simulink model "dt_crff2_non_ideal"  (R2025b)
settings: Solver=VariableStepAuto  StartTime=0.0  StopTime=10.0  RelTol=1e-3
undefined symbols (not defined in the file): Fs, k01, K01, k02, K02, k03, K03, k04, K04, k05, K05, k06, K06, k07, K07, k08, K08, k09, K09, k10, K10, k11, K11, k12, K12, k13, K13, k14, K14, k15, K15, k16, K16, k17, K17, k18, K18, k19, K19, k20, K20, k21, K21, k22, K22, k23, K23, k24, K24, k25, K25, k26, K26, k27, K27, k28, K28, k29, K29, k30 ... (+66)
libraries: msbAdcMeasurements x1, cstblocks x1, dspobslib x1
settings Model: Creator=divya  LastModifiedBy=divya

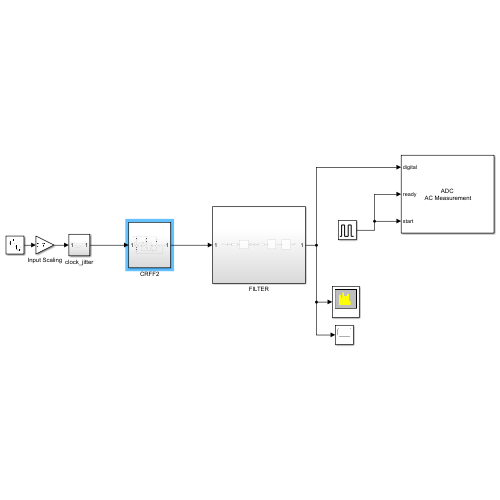
[thumbnail: Simulink's stored preview of the top-level diagram]
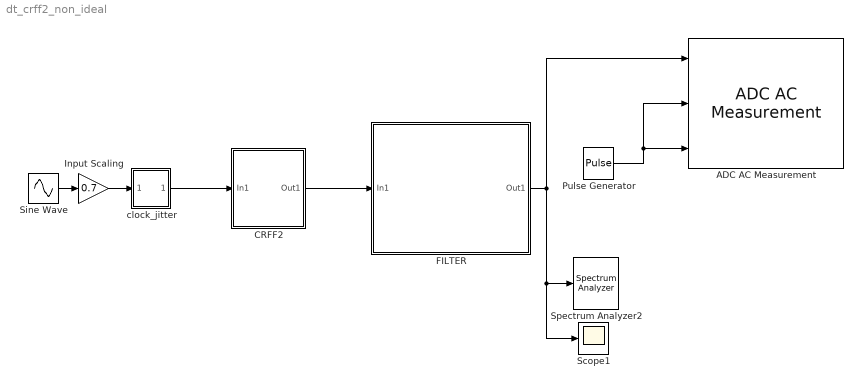
== system dt_crff2_non_ideal ==
  ADC AC Measurement : msbAdcMeasurements/ADC AC Measurement  DistortionMeasurement=Harmonic  InputFrequency=100  Method=Filter bank (slower, requires extra simulation time)  RBW=0.48828  AutoSetRBW=on  NBits=18  Frequency=512e3/1024  HoldOffTime=0  OutputToWorkspace=on  VariableName=adc_ac_out  ShowSpectrum=on
      link override ADC AC Measurement/ADC AC Measurement Spectrum Analyzer: YLimits=[-1125000 -875000]
  CRFF2 : Subsystem
  FILTER : Subsystem
  Input Scaling : Gain  Gain=0.7
  Pulse Generator : DiscretePulseGenerator  PulseType=Time based  Period=1/1e3  PulseWidth=50
  Scope1 : Scope
      settings: ActiveDisplayYMinimum=-1.8E-8  ActiveDisplayYMaximum=1.8E-8
  Sine Wave : Sin  Amplitude=0.5  Frequency=628  SampleTime=1/512e3
  Spectrum Analyzer2 : SpectrumAnalyzer  WindowPosition=[1.000000,1.000000,1536.000000,841.000000,]  ScopeFrameLocation=window  PlotAsTwoSidedSpectrum=off  YLimits=[-207.6433 -122.1238]  SelectedToolstripTab=spectrumAnalyzerToolstrip.spectrumTab
  clock_jitter : Subsystem
  wires:
  CRFF2/1(Out1) -> FILTER/1(In1)
  clock_jitter/1(Out1) -> CRFF2/1(In1)
  Pulse Generator/1 -> ADC AC Measurement/3, ADC AC Measurement/2
  Input Scaling/1 -> clock_jitter/1(In1)
  FILTER/1(Out1) -> ADC AC Measurement/1, Scope1/1, Spectrum Analyzer2/1
  Sine Wave/1 -> Input Scaling/1

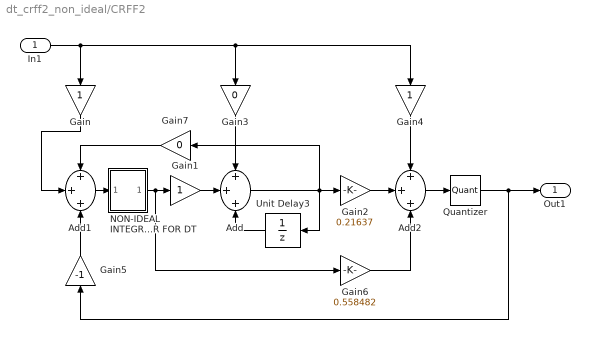
== system dt_crff2_non_ideal/CRFF2 ==
  In1 : Inport
  Add : Sum  RequirementInfo={} %GIDa_3c5f622a_b94f_44a6_8cf5_4d620276e7c1  Inputs=+++
  Add1 : Sum  RequirementInfo={} %GIDa_2560f21a_28c6_47ea_a0df_4ad0b40fcbe5  Inputs=+++
  Add2 : Sum  RequirementInfo={} %GIDa_8d62e077_71f1_449a_b76b_2bda6cdf909d  Inputs=+++
  Gain : Gain  RequirementInfo={} %GIDa_ad436a21_f5dd_4e55_a482_890f0f126b90
  Gain1 : Gain  RequirementInfo={} %GIDa_c3b20c88_4060_4312_8646_d3b95ed7ab58
  Gain2 : Gain  RequirementInfo={} %GIDa_e70bd45e_24a6_44be_901f_827768984ba0  Gain=0.21637
  Gain3 : Gain  RequirementInfo={} %GIDa_dd2b615f_3e17_4946_afe5_8b8154edc31d  Gain=0
  Gain4 : Gain  RequirementInfo={} %GIDa_6be3646e_fc84_4f83_a120_e64b39dc9dcc
  Gain5 : Gain  RequirementInfo={} %GIDa_626d9d2e_4885_4ec0_a1ca_3018a1e5cf17  Gain=-1
  Gain6 : Gain  RequirementInfo={} %GIDa_3141b0aa_4885_4fd5_b8bf_797217bb3f0f  Gain=0.558482
  Gain7 : Gain  RequirementInfo={} %GIDa_7d31512d_d1b8_464e_a954_aed416029a99  Gain=0
  NON-IDEAL INTEGRATOR FOR DT : Subsystem
  Quantizer : Quantizer  RequirementInfo={} %GIDa_4572926b_fdfc_440d_bb41_09360aa605ce  QuantizationInterval=0.25
  Unit Delay3 : UnitDelay  SampleTime=1/(48e3*64)  HasFrameUpgradeWarning=on
  Out1 : Outport
  wires:
  Gain4/1 -> Add2/1
  Gain1/1 -> Add/2
  Add1/1 -> NON-IDEAL INTEGRATOR FOR DT/1(In2)
  Gain3/1 -> Add/1
  Gain5/1 -> Add1/3
  Gain2/1 -> Add2/2
  Unit Delay3/1 -> Add/3
  Gain7/1 -> Add1/1
  Quantizer/1 -> Out1/1, Gain5/1
  Add2/1 -> Quantizer/1
  Add/1 -> Unit Delay3/1, Gain7/1, Gain2/1
  In1/1 -> Gain/1, Gain3/1, Gain4/1
  NON-IDEAL INTEGRATOR FOR DT/1(Out1) -> Gain6/1, Gain1/1
  Gain6/1 -> Add2/3
  Gain/1 -> Add1/2

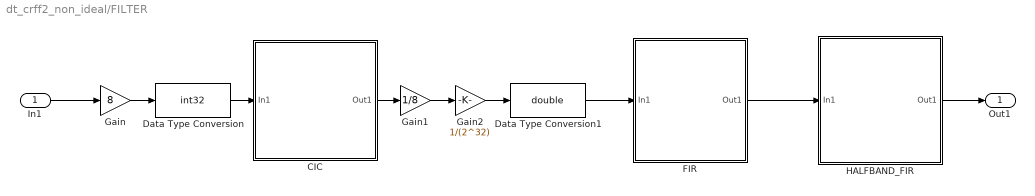
== system dt_crff2_non_ideal/FILTER ==
  In1 : Inport
  CIC : Subsystem
  Data Type Conversion : DataTypeConversion  OutDataTypeStr=int32  SaturateOnIntegerOverflow=off  RndMeth=Floor
  Data Type Conversion1 : DataTypeConversion  OutDataTypeStr=double  SaturateOnIntegerOverflow=off  RndMeth=Floor
  FIR : Subsystem
  Gain : Gain  Gain=8
  Gain1 : Gain  Gain=1/8
  Gain2 : Gain  Gain=1/(2^32)
  HALFBAND_FIR : Subsystem
  Out1 : Outport
  wires:
  Gain2/1 -> Data Type Conversion1/1
  Gain1/1 -> Gain2/1
  Data Type Conversion/1 -> CIC/1(In1)
  CIC/1(Out1) -> Gain1/1
  Gain/1 -> Data Type Conversion/1
  FIR/1(Out1) -> HALFBAND_FIR/1(In1)
  In1/1 -> Gain/1
  Data Type Conversion1/1 -> FIR/1(In1)
  HALFBAND_FIR/1(Out1) -> Out1/1

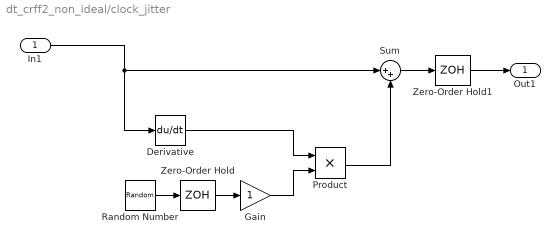
== system dt_crff2_non_ideal/clock_jitter ==
  In1 : Inport
  Derivative : Derivative
  Gain : Gain
  Product : Product
  Random Number : RandomNumber  SampleTime=0.1
  Sum : Sum  Inputs=|++
  Zero-Order Hold : ZeroOrderHold  SampleTime=-1
  Zero-Order Hold1 : ZeroOrderHold  SampleTime=-1
  Out1 : Outport
  wires:
  In1/1 -> Derivative/1, Sum/1
  Derivative/1 -> Product/1
  Zero-Order Hold1/1 -> Out1/1
  Sum/1 -> Zero-Order Hold1/1
  Random Number/1 -> Zero-Order Hold/1
  Product/1 -> Sum/2
  Zero-Order Hold/1 -> Gain/1
  Gain/1 -> Product/2

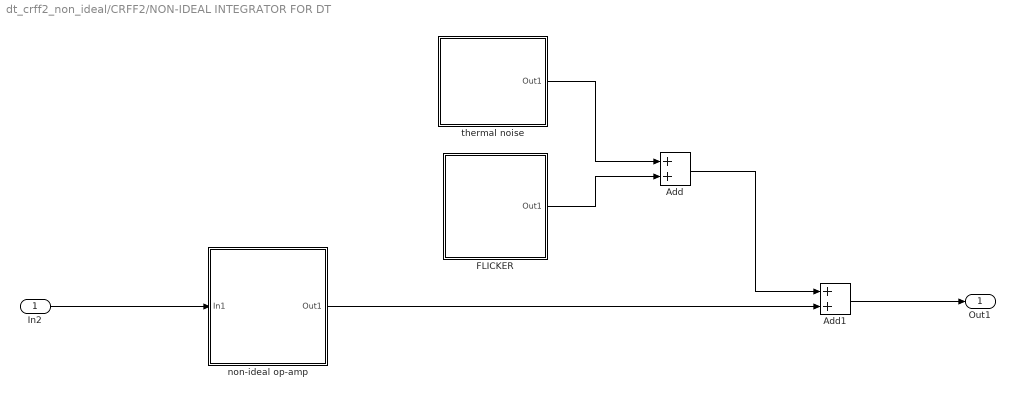
== system dt_crff2_non_ideal/CRFF2/NON-IDEAL INTEGRATOR FOR DT ==
  In2 : Inport
  Add : Sum
  Add1 : Sum
  FLICKER : Subsystem
  "non-ideal op-amp " : Subsystem
  thermal noise : Subsystem
  Out1 : Outport
  wires:
  In2/1 -> "non-ideal op-amp "/1(In1)
  Add/1 -> Add1/1
  Add1/1 -> Out1/1
  "non-ideal op-amp "/1(Out1) -> Add1/2
  thermal noise/1(Out1) -> Add/1
  FLICKER/1(Out1) -> Add/2

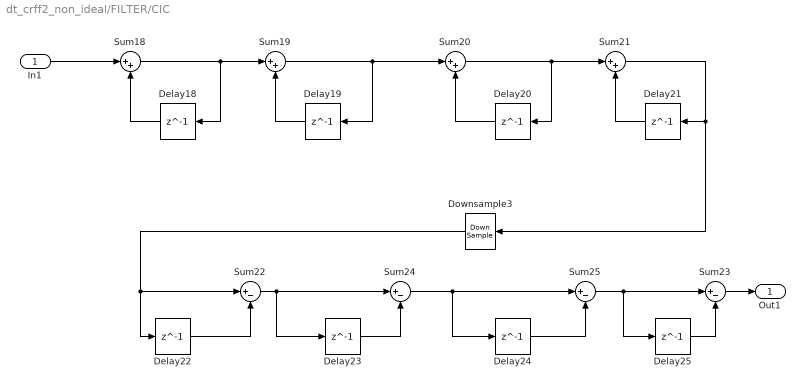
== system dt_crff2_non_ideal/FILTER/CIC ==
  In1 : Inport
  Delay{18..25} (8 alike) : Delay  DelayLength=1  InputProcessing=Columns as channels (frame based)
  Downsample3 : DownSample  N=128  RateOptions=Allow multirate processing
  Sum{18..21} (4 alike) : Sum  Inputs=|++
  Sum{22..25} (4 alike) : Sum  Inputs=|+-
  Out1 : Outport
  wires:
  Downsample3/1 -> Sum22/1, Delay22/1
  Sum19/1 -> Delay19/1, Sum20/1
  Sum20/1 -> Delay20/1, Sum21/1
  Sum22/1 -> Delay23/1, Sum24/1
  Delay24/1 -> Sum25/2
  Sum24/1 -> Delay24/1, Sum25/1
  In1/1 -> Sum18/1
  Sum18/1 -> Delay18/1, Sum19/1
  Delay18/1 -> Sum18/2
  Sum25/1 -> Delay25/1, Sum23/1
  Delay20/1 -> Sum20/2
  Delay22/1 -> Sum22/2
  Delay21/1 -> Sum21/2
  Sum21/1 -> Downsample3/1, Delay21/1
  Delay23/1 -> Sum24/2
  Delay19/1 -> Sum19/2
  Delay25/1 -> Sum23/2
  Sum23/1 -> Out1/1

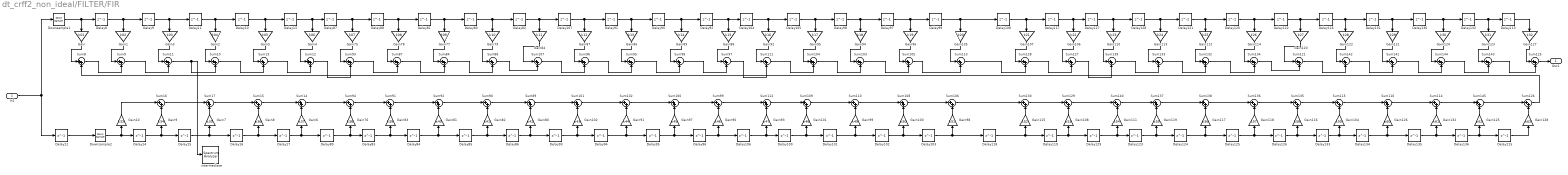
== system dt_crff2_non_ideal/FILTER/FIR ==
  In1 : Inport
  Delay{8..17,80..108,113,115..136} (62 alike) : Delay  DelayLength=1  InputProcessing=Columns as channels (frame based)
  Downsample1 : DownSample  N=4  RateOptions=Allow multirate processing
  Downsample2 : DownSample  N=4  RateOptions=Allow multirate processing
  Gain : Gain  Gain=k01
  Gain1 : Gain  Gain=k02
  Gain10 : Gain  Gain=k33
  Gain100 : Gain  Gain=k50
  Gain101 : Gain  Gain=k48
  Gain102 : Gain  Gain=k43
  Gain104 : Gain  Gain=k59
  Gain105 : Gain  Gain=k20
  Gain106 : Gain  Gain=k22
  Gain107 : Gain  Gain=k21
  Gain108 : Gain  Gain=k53
  Gain110 : Gain  Gain=k23
  Gain111 : Gain  Gain=k54
  Gain112 : Gain  Gain=k25
  Gain113 : Gain  Gain=k24
  Gain114 : Gain  Gain=k26
  Gain115 : Gain  Gain=k52
  Gain116 : Gain  Gain=k58
  Gain117 : Gain  Gain=k56
  Gain118 : Gain  Gain=k57
  Gain119 : Gain  Gain=k55
  Gain120 : Gain  Gain=k27
  Gain121 : Gain  Gain=k29
  Gain122 : Gain  Gain=k28
  Gain123 : Gain  Gain=k31
  Gain124 : Gain  Gain=k30
  Gain125 : Gain  Gain=k62
  Gain126 : Gain  Gain=k60
  Gain127 : Gain  Gain=k32
  Gain128 : Gain  Gain=k63
  Gain132 : Gain  Gain=k61
  Gain2 : Gain  Gain=k04
  Gain3 : Gain  Gain=k03
  Gain4 : Gain  Gain=k06
  Gain5 : Gain  Gain=k05
  Gain6 : Gain  Gain=k37
  Gain7 : Gain  Gain=k35
  Gain75 : Gain  Gain=k07
  Gain76 : Gain  Gain=k38
  Gain77 : Gain  Gain=k09
  Gain78 : Gain  Gain=k08
  Gain79 : Gain  Gain=k10
  Gain8 : Gain  Gain=k36
  Gain80 : Gain  Gain=k42
  Gain81 : Gain  Gain=k40
  Gain82 : Gain  Gain=k41
  Gain83 : Gain  Gain=k39
  Gain84 : Gain  Gain=k11
  Gain86 : Gain  Gain=k13
  Gain87 : Gain  Gain=k12
  Gain88 : Gain  Gain=k15
  Gain89 : Gain  Gain=k14
  Gain9 : Gain  Gain=k34
  Gain90 : Gain  Gain=k46
  Gain91 : Gain  Gain=k44
  Gain92 : Gain  Gain=k16
  Gain93 : Gain  Gain=k47
  Gain94 : Gain  Gain=k18
  Gain95 : Gain  Gain=k17
  Gain96 : Gain  Gain=k19
  Gain97 : Gain  Gain=k45
  Gain98 : Gain  Gain=k51
  Gain99 : Gain  Gain=k49
  Sum{8..17,84,87..116,121,125..130,132..145} (62 alike) : Sum  Inputs=|++
  intermediate : SpectrumAnalyzer  WindowPosition=[1.000000,1.000000,1536.000000,841.000000,]  ScopeFrameLocation=window  Span=1000  StartFrequency=-500  StopFrequency=500  YLimits=[-211.6942 -128.1697]
  Out1 : Outport
  wires:
  Sum107/1 -> Sum96/2
  Delay104/1 -> Delay105/1, Gain92/1
  Delay88/1 -> Gain78/1, Delay81/1
  Sum98/1 -> Sum97/2
  Gain132/1 -> Sum114/2
  Sum135/1 -> Sum115/1
  Downsample1/1 -> Delay8/1, Gain/1
  Gain80/1 -> Sum89/2
  Delay84/1 -> Delay85/1, Gain81/1
  Gain120/1 -> Sum121/1
  Sum142/1 -> Sum141/2
  Sum96/1 -> Sum95/2
  Delay108/1 -> Gain107/1, Delay117/1
  Delay92/1 -> Delay104/1, Gain88/1
  Sum100/1 -> Sum99/1
  Sum94/1 -> Sum91/1
  Delay129/1 -> Gain111/1, Delay123/1
  Gain116/1 -> Sum135/2
  Delay81/1 -> Delay80/1, Gain77/1
  Delay132/1 -> Delay113/1, Gain123/1
  Delay101/1 -> Delay102/1, Gain99/1
  Sum137/1 -> Sum138/1
  Gain96/1 -> Sum105/1
  Delay125/1 -> Gain118/1, Delay126/1
  Delay116/1 -> Delay131/1, Gain122/1
  Delay97/1 -> Gain96/1, Delay99/1
  Downsample2/1 -> Gain10/1, Delay14/1
  Delay80/1 -> Delay82/1, Gain79/1
  Gain111/1 -> Sum140/2
  Gain2/1 -> Sum10/1
  Sum17/1 -> Sum15/1
  Gain118/1 -> Sum136/2
  Delay89/1 -> Gain76/1, Delay83/1
  Sum126/1 -> Sum8/2
  Gain123/1 -> Sum143/1
  Delay113/1 -> Gain127/1
  Sum92/1 -> Sum90/1
  Gain100/1 -> Sum108/2
  Sum10/1 -> Sum13/2
  Gain3/1 -> Sum11/1
  Delay122/1 -> Gain120/1, Delay116/1
  Sum116/1 -> Sum114/1
  Delay124/1 -> Delay125/1, Gain117/1
  Gain127/1 -> Sum125/1
  Delay121/1 -> Delay120/1, Gain112/1
  Gain94/1 -> Sum103/1
  Delay117/1 -> Delay127/1, Gain106/1
  Sum9/1 -> Sum11/2
  Delay91/1 -> Delay90/1, Gain86/1
  Sum13/1 -> Sum12/2
  Delay11/1 -> Delay10/1, Gain2/1
  Delay99/1 -> Gain105/1, Delay108/1
  Gain87/1 -> Sum96/1
  Gain97/1 -> Sum100/2
  Gain90/1 -> Sum99/2
  Delay135/1 -> Gain132/1, Delay136/1
  Gain119/1 -> Sum137/2
  Gain126/1 -> Sum116/2
  Delay9/1 -> Gain3/1, Delay11/1
  Sum97/1 -> Sum111/2
  Sum129/1 -> Sum140/1
  Gain105/1 -> Sum113/1
  Delay82/1 -> Gain84/1, Delay107/1
  Gain5/1 -> Sum13/1
  Delay10/1 -> Gain5/1, Delay13/1
  Delay118/1 -> Gain115/1, Delay119/1
  Sum144/1 -> Sum143/2
  Delay127/1 -> Delay128/1, Gain110/1
  Gain84/1 -> Sum107/1
  Sum127/1 -> Sum139/2
  Sum106/1 -> Sum130/1
  Delay123/1 -> Gain119/1, Delay124/1
  Sum103/1 -> Sum105/2
  Delay14/1 -> Gain9/1, Delay15/1
  Delay100/1 -> Gain101/1, Delay101/1
  Sum87/1 -> Sum84/2
  Sum141/1 -> Sum144/2
  Sum128/1 -> Sum127/2
  Delay130/1 -> Gain124/1, Delay132/1
  Sum108/1 -> Sum106/1
  Sum140/1 -> Sum137/1
  Gain114/1 -> Sum134/1
  Delay119/1 -> Delay129/1, Gain108/1
  Gain107/1 -> Sum128/1
  Gain1/1 -> Sum9/1
  Delay86/1 -> Delay93/1, Gain80/1
  Gain10/1 -> Sum16/1
  Delay136/1 -> Delay115/1, Gain125/1
  Gain98/1 -> Sum106/2
  Sum93/1 -> Sum87/2
  Sum88/1 -> Sum107/2
  Gain110/1 -> Sum139/1
  Delay8/1 -> Delay9/1, Gain1/1
  Gain9/1 -> Sum16/2
  Sum133/1 -> Sum132/2
  Delay93/1 -> Gain102/1, Delay94/1
  Delay126/1 -> Delay133/1, Gain116/1
  In1/1 -> Delay12/1, Downsample1/1
  Delay12/1 -> Downsample2/1
  Gain106/1 -> Sum127/1
  Delay96/1 -> Delay106/1, Gain90/1
  Sum115/1 -> Sum116/1
  Delay106/1 -> Gain93/1, Delay100/1
  Sum109/1 -> Sum110/1
  Sum138/1 -> Sum136/1
  Sum101/1 -> Sum102/1
  Gain77/1 -> Sum84/1
  Sum130/1 -> Sum129/1
  Gain88/1 -> Sum97/1
  Delay120/1 -> Delay122/1, Gain114/1
  Gain115/1 -> Sum130/2
  Gain83/1 -> Sum91/2
  Delay131/1 -> Delay130/1, Gain121/1
  Gain/1 -> Sum8/1
  Gain95/1 -> Sum104/1
  Delay133/1 -> Gain104/1, Delay134/1
  Sum136/1 -> Sum135/1
  Delay94/1 -> Delay95/1, Gain91/1
  Sum112/1 -> Sum109/1
  Sum12/1 -> Sum93/2
  Sum113/1 -> Sum128/2
  Sum104/1 -> Sum103/2
  Gain89/1 -> Sum98/1
  Delay17/1 -> Delay89/1, Gain6/1
  Sum134/1 -> Sum121/2
  Sum121/1 -> Sum142/2
  Gain91/1 -> Sum102/2
  Sum105/1 -> Sum113/2
  Gain4/1 -> Sum12/1
  Gain82/1 -> Sum90/2
  Gain122/1 -> Sum142/1
  Delay134/1 -> Delay135/1, Gain126/1
  Delay105/1 -> Gain95/1, Delay98/1
  Delay15/1 -> Delay16/1, Gain7/1
  Sum132/1 -> Sum134/2
  Gain8/1 -> Sum15/2
  Gain86/1 -> Sum95/1
  Delay85/1 -> Gain82/1, Delay86/1
  Sum89/1 -> Sum101/1
  Gain121/1 -> Sum141/1
  Delay102/1 -> Gain100/1, Delay103/1
  Gain75/1 -> Sum93/1
  Gain102/1 -> Sum101/2
  Sum16/1 -> Sum17/1
  Sum91/1 -> Sum92/1
  Gain99/1 -> Sum110/2
  Gain7/1 -> Sum17/2
  Sum114/1 -> Sum145/1
  Delay87/1 -> Delay88/1, Gain75/1
  Gain78/1 -> Sum87/1
  Gain117/1 -> Sum138/2
  Delay107/1 -> Delay91/1, Gain87/1
  Gain76/1 -> Sum94/2
  Gain92/1 -> Sum111/1
  Delay16/1 -> Gain8/1, Delay17/1
  Delay98/1 -> Delay97/1, Gain94/1
  Delay95/1 -> Gain97/1, Delay96/1
  Gain104/1 -> Sum115/2
  Sum84/1 -> Sum88/2
  Sum11/1 -> intermediate/1, Sum10/2
  Sum111/1 -> Sum104/2
  Delay90/1 -> Gain89/1, Delay92/1
  Sum14/1 -> Sum94/1
  Sum143/1 -> Sum125/2
  Delay13/1 -> Delay87/1, Gain4/1
  Gain101/1 -> Sum109/2
  Gain81/1 -> Sum92/2
  Gain112/1 -> Sum132/1
  Delay103/1 -> Delay118/1, Gain98/1
  Sum95/1 -> Sum98/2
  Gain125/1 -> Sum145/2
  Gain79/1 -> Sum88/1
  Sum99/1 -> Sum112/1
  Sum145/1 -> Sum126/1
  Gain113/1 -> Sum133/1
  Sum8/1 -> Sum9/2
  Sum110/1 -> Sum108/1
  Sum90/1 -> Sum89/1
  Sum139/1 -> Sum133/2
  Delay83/1 -> Gain83/1, Delay84/1
  Delay128/1 -> Gain113/1, Delay121/1
  Gain6/1 -> Sum14/2
  Sum125/1 -> Out1/1
  Gain93/1 -> Sum112/2
  Sum15/1 -> Sum14/1
  Gain108/1 -> Sum129/2
  Gain128/1 -> Sum126/2
  Delay115/1 -> Gain128/1
  Gain124/1 -> Sum144/1
  Sum102/1 -> Sum100/1

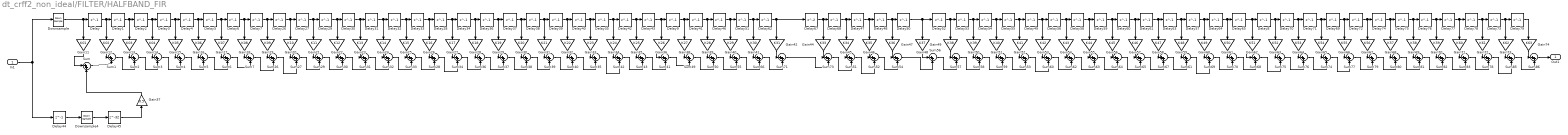
== system dt_crff2_non_ideal/FILTER/HALFBAND_FIR ==
  In1 : Inport
  Delay{,1..9,26..44,46..65,68..79} (61 alike) : Delay  DelayLength=1  InputProcessing=Columns as channels (frame based)
  Delay45 : Delay  DelayLength=32  InputProcessing=Columns as channels (frame based)
  Delay67 : Delay  InputProcessing=Columns as channels (frame based)
  Downsample : DownSample  RateOptions=Allow multirate processing
  Downsample4 : DownSample  RateOptions=Allow multirate processing
  Gain11 : Gain  Gain=K01
  Gain12 : Gain  Gain=K02
  Gain13 : Gain  Gain=K03
  Gain14 : Gain  Gain=K04
  Gain15 : Gain  Gain=K05
  Gain16 : Gain  Gain=K06
  Gain17 : Gain  Gain=K07
  Gain18 : Gain  Gain=K08
  Gain19 : Gain  Gain=K09
  Gain20 : Gain  Gain=K10
  Gain21 : Gain  Gain=K11
  Gain22 : Gain  Gain=K12
  Gain23 : Gain  Gain=K13
  Gain24 : Gain  Gain=K14
  Gain25 : Gain  Gain=K15
  Gain26 : Gain  Gain=K16
  Gain27 : Gain  Gain=K17
  Gain28 : Gain  Gain=K18
  Gain29 : Gain  Gain=K19
  Gain30 : Gain  Gain=K20
  Gain31 : Gain  Gain=K21
  Gain32 : Gain  Gain=K22
  Gain33 : Gain  Gain=K23
  Gain34 : Gain  Gain=K24
  Gain35 : Gain  Gain=K25
  Gain36 : Gain  Gain=K26
  Gain37 : Gain  Gain=0.5
  Gain38 : Gain  Gain=K27
  Gain39 : Gain  Gain=K28
  Gain40 : Gain  Gain=K29
  Gain41 : Gain  Gain=K30
  Gain42 : Gain  Gain=K31
  Gain44 : Gain  Gain=K33
  Gain45 : Gain  Gain=K34
  Gain46 : Gain  Gain=K35
  Gain47 : Gain  Gain=K36
  Gain48 : Gain  Gain=K37
  Gain49 : Gain  Gain=K38
  Gain50 : Gain  Gain=K39
  Gain51 : Gain  Gain=K40
  Gain52 : Gain  Gain=K41
  Gain53 : Gain  Gain=K42
  Gain54 : Gain  Gain=K43
  Gain55 : Gain  Gain=K44
  Gain56 : Gain  Gain=K45
  Gain57 : Gain  Gain=K46
  Gain58 : Gain  Gain=K47
  Gain59 : Gain  Gain=K48
  Gain60 : Gain  Gain=K49
  Gain61 : Gain  Gain=K50
  Gain62 : Gain  Gain=K51
  Gain63 : Gain  Gain=K52
  Gain64 : Gain  Gain=K53
  Gain65 : Gain  Gain=K54
  Gain66 : Gain  Gain=K55
  Gain67 : Gain  Gain=K56
  Gain68 : Gain  Gain=K57
  Gain69 : Gain  Gain=K58
  Gain70 : Gain  Gain=K59
  Gain71 : Gain  Gain=K60
  Gain72 : Gain  Gain=K61
  Gain73 : Gain  Gain=K62
  Gain74 : Gain  Gain=K63
  Sum{,1..7,26..43,49..71,73..83,85..86} (62 alike) : Sum  Inputs=|++
  Out1 : Outport
  wires:
  Gain31/1 -> Sum39/1
  Delay30/1 -> Delay31/1, Gain23/1
  Gain55/1 -> Sum63/1
  Delay40/1 -> Delay35/1, Gain33/1
  Delay31/1 -> Delay32/1, Gain24/1
  Gain46/1 -> Sum52/1
  Gain30/1 -> Sum38/1
  Delay53/1 -> Delay54/1, Gain50/1
  Downsample/1 -> Gain11/1, Delay/1
  Delay47/1 -> Delay48/1, Gain46/1
  Sum35/1 -> Sum42/2
  Delay71/1 -> Delay69/1, Gain65/1
  Gain68/1 -> Sum80/1
  Delay5/1 -> Delay6/1, Gain17/1
  Delay59/1 -> Delay60/1, Gain56/1
  Sum2/1 -> Sum3/2
  Gain22/1 -> Sum30/1
  Sum27/1 -> Sum29/2
  Gain53/1 -> Sum60/1
  Sum63/1 -> Sum64/2
  Sum65/1 -> Sum67/2
  Delay38/1 -> Delay39/1, Gain31/1
  Delay4/1 -> Delay5/1, Gain16/1
  Sum78/1 -> Sum85/2
  Delay45/1 -> Gain37/1
  Sum7/1 -> Sum26/2
  Delay50/1 -> Delay52/1, Gain48/1
  Gain13/1 -> Sum2/1
  Sum62/1 -> Sum63/2
  Delay49/1 -> Delay56/1, Gain53/1
  Delay62/1 -> Delay67/1, Gain42/1
  Gain24/1 -> Sum32/1
  Gain61/1 -> Sum70/1
  Delay7/1 -> Delay26/1, Gain19/1
  Delay55/1 -> Delay49/1, Gain52/1
  Delay3/1 -> Delay4/1, Gain15/1
  Gain36/1 -> Sum41/1
  Gain56/1 -> Sum64/1
  Sum34/1 -> Sum36/2
  Sum70/1 -> Sum68/2
  Gain52/1 -> Sum53/1
  Delay77/1 -> Delay78/1, Gain71/1
  Delay34/1 -> Delay36/1, Gain28/1
  Delay79/1 -> Gain74/1
  Delay32/1 -> Delay33/1, Gain25/1
  Delay1/1 -> Delay2/1, Gain13/1
  Gain20/1 -> Sum27/1
  Gain49/1 -> Sum57/1
  Gain50/1 -> Sum58/1
  Delay65/1 -> Delay8/1, Gain62/1
  In1/1 -> Downsample/1, Delay44/1
  Delay42/1 -> Delay43/1, Gain35/1
  Gain16/1 -> Sum5/1
  Sum74/1 -> Sum77/2
  Sum50/1 -> Sum55/2
  Gain42/1 -> Sum71/1
  Sum43/1 -> Sum41/2
  Sum77/1 -> Sum79/2
  Delay67/1 -> Delay68/1, Gain44/1
  Sum1/1 -> Sum2/2
  Gain35/1 -> Sum43/1
  Sum31/1 -> Sum32/2
  Delay2/1 -> Delay3/1, Gain14/1
  Delay52/1 -> Delay53/1, Gain49/1
  Delay39/1 -> Delay40/1, Gain32/1
  Delay48/1 -> Delay50/1, Gain47/1
  Gain74/1 -> Sum86/1
  Delay60/1 -> Delay61/1, Gain57/1
  Delay26/1 -> Delay27/1, Gain20/1
  Sum58/1 -> Sum59/2
  Sum68/1 -> Sum75/2
  Gain32/1 -> Sum40/1
  Sum/1 -> Sum1/2
  Sum59/1 -> Sum53/2
  Delay51/1 -> Delay62/1, Gain41/1
  Sum38/1 -> Sum39/2
  Sum67/1 -> Sum61/2
  Delay74/1 -> Delay75/1, Gain68/1
  Gain26/1 -> Sum28/1
  Gain63/1 -> Sum75/1
  Delay6/1 -> Delay7/1, Gain18/1
  Sum71/1 -> Sum73/2
  Sum82/1 -> Sum83/2
  Delay28/1 -> Delay34/1, Gain27/1
  Sum56/1 -> Sum57/2
  Gain73/1 -> Sum85/1
  Gain47/1 -> Sum54/1
  Delay57/1 -> Delay64/1, Gain60/1
  Delay35/1 -> Delay42/1, Gain34/1
  Gain45/1 -> Sum51/1
  Delay36/1 -> Delay37/1, Gain29/1
  Gain57/1 -> Sum65/1
  Sum41/1 -> Sum49/2
  Sum76/1 -> Sum74/2
  Delay64/1 -> Delay65/1, Gain61/1
  Sum39/1 -> Sum40/2
  Gain34/1 -> Sum42/1
  Delay69/1 -> Delay72/1, Gain66/1
  Delay/1 -> Delay1/1, Gain12/1
  Gain44/1 -> Sum73/1
  Sum6/1 -> Sum7/2
  Gain14/1 -> Sum3/1
  Gain58/1 -> Sum67/1
  Sum3/1 -> Sum4/2
  Delay63/1 -> Delay57/1, Gain59/1
  Sum40/1 -> Sum35/2
  Gain19/1 -> Sum26/1
  Gain54/1 -> Sum62/1
  Sum57/1 -> Sum58/2
  Sum26/1 -> Sum27/2
  Sum75/1 -> Sum76/2
  Gain12/1 -> Sum1/1
  Sum54/1 -> Sum56/2
  Delay75/1 -> Delay76/1, Gain69/1
  Gain66/1 -> Sum77/1
  Sum64/1 -> Sum65/2
  Gain70/1 -> Sum82/1
  Sum79/1 -> Sum80/2
  Gain21/1 -> Sum29/1
  Sum81/1 -> Sum82/2
  Gain48/1 -> Sum56/1
  Downsample4/1 -> Delay45/1
  Delay70/1 -> Delay71/1, Gain64/1
  Sum60/1 -> Sum62/2
  Delay46/1 -> Delay51/1, Gain40/1
  Sum53/1 -> Sum60/2
  Gain38/1 -> Sum49/1
  Gain23/1 -> Sum31/1
  Gain18/1 -> Sum7/1
  Sum73/1 -> Sum51/2
  Sum66/1 -> Sum71/2
  Gain25/1 -> Sum33/1
  Gain17/1 -> Sum6/1
  Delay29/1 -> Delay30/1, Gain22/1
  Delay44/1 -> Downsample4/1
  Gain72/1 -> Sum78/1
  Delay33/1 -> Delay28/1, Gain26/1
  Sum55/1 -> Sum66/2
  Sum42/1 -> Sum43/2
  Sum86/1 -> Out1/1
  Sum80/1 -> Sum81/2
  Delay72/1 -> Delay74/1, Gain67/1
  Delay37/1 -> Delay38/1, Gain30/1
  Delay68/1 -> Delay47/1, Gain45/1
  Gain15/1 -> Sum4/1
  Delay58/1 -> Delay59/1, Gain55/1
  Delay56/1 -> Delay58/1, Gain54/1
  Sum28/1 -> Sum34/2
  Gain29/1 -> Sum37/1
  Sum33/1 -> Sum28/2
  Gain71/1 -> Sum83/1
  Gain41/1 -> Sum66/1
  Sum83/1 -> Sum78/2
  Sum32/1 -> Sum33/2
  Gain39/1 -> Sum50/1
  Sum61/1 -> Sum69/2
  Sum36/1 -> Sum37/2
  Sum69/1 -> Sum70/2
  Gain40/1 -> Sum55/1
  Gain69/1 -> Sum81/1
  Gain62/1 -> Sum68/1
  Delay54/1 -> Delay55/1, Gain51/1
  Gain67/1 -> Sum79/1
  Sum52/1 -> Sum54/2
  Delay27/1 -> Delay29/1, Gain21/1
  Sum29/1 -> Sum30/2
  Gain59/1 -> Sum61/1
  Gain33/1 -> Sum35/1
  Gain64/1 -> Sum76/1
  Delay61/1 -> Delay63/1, Gain58/1
  Delay43/1 -> Delay9/1, Gain36/1
  Gain11/1 -> Sum/1
  Sum5/1 -> Sum6/2
  Sum30/1 -> Sum31/2
  Gain65/1 -> Sum74/1
  Delay73/1 -> Delay79/1, Gain73/1
  Delay41/1 -> Delay46/1, Gain39/1
  Sum51/1 -> Sum52/2
  Gain27/1 -> Sum34/1
  Sum37/1 -> Sum38/2
  Gain37/1 -> Sum/2
  Sum4/1 -> Sum5/2
  Delay76/1 -> Delay77/1, Gain70/1
  Gain28/1 -> Sum36/1
  Gain51/1 -> Sum59/1
  Delay78/1 -> Delay73/1, Gain72/1
  Sum49/1 -> Sum50/2
  Sum85/1 -> Sum86/2
  Gain60/1 -> Sum69/1
  Delay8/1 -> Delay70/1, Gain63/1
  Delay9/1 -> Gain38/1, Delay41/1

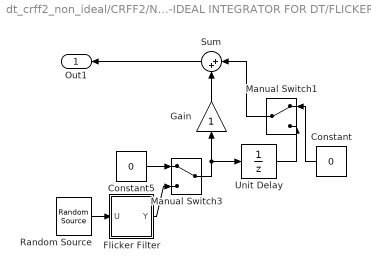
== system dt_crff2_non_ideal/CRFF2/NON-IDEAL INTEGRATOR FOR DT/FLICKER ==
  Constant : Constant  Value=0
  Constant5 : Constant  Value=0  SampleTime=1/Fs
  Flicker Filter : Subsystem
  Gain : Gain
  Manual Switch1 : ManualSwitch
  Manual Switch3 : ManualSwitch
  Random Source : dspobslib/Random Source  SrcType=Gaussian  NormMethod=Ziggurat  CltLength=12  MinVal=0  MaxVal=1  MeanVal=0  VarVal=1  RepMode=Not repeatable  rawSeed=1  IsInherit=off  SampMode=Discrete  SampTime=1/Fs  SampFrame=1  DataType=Double  OutComplex=Real  OutputFrames=off
  Sum : Sum  Inputs=|++
  Unit Delay : UnitDelay  SampleTime=1/Fs  HasFrameUpgradeWarning=on
  Out1 : Outport
  wires:
  Manual Switch3/1 -> Gain/1, Unit Delay/1
  Random Source/1 -> Flicker Filter/1(U)
  Unit Delay/1 -> Manual Switch1/2
  Constant5/1 -> Manual Switch3/1
  Constant/1 -> Manual Switch1/1
  Gain/1 -> Sum/2
  Manual Switch1/1 -> Sum/1
  Flicker Filter/1(Y) -> Manual Switch3/2
  Sum/1 -> Out1/1

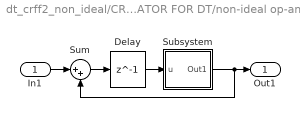
== system dt_crff2_non_ideal/CRFF2/NON-IDEAL INTEGRATOR FOR DT/non-ideal op-amp  ==
  In1 : Inport
  Delay : Delay  DelayLength=1  InputProcessing=Columns as channels (frame based)  SampleTime=1/(2e3*128)
  Subsystem : Subsystem
  Sum : Sum  Inputs=|++
  Out1 : Outport
  wires:
  Subsystem/1(Out1) -> Out1/1, Sum/2
  In1/1 -> Sum/1
  Sum/1 -> Delay/1
  Delay/1 -> Subsystem/1(u)

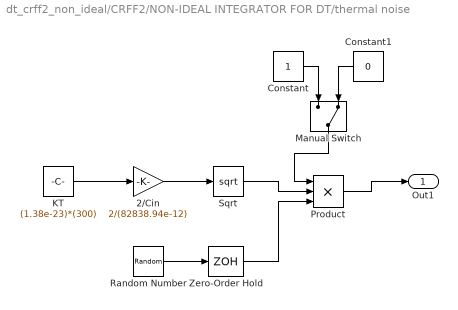
== system dt_crff2_non_ideal/CRFF2/NON-IDEAL INTEGRATOR FOR DT/thermal noise ==
  2/Cin : Gain  Gain=2/(82838.94e-12)
  Constant : Constant
  Constant1 : Constant  Value=0
  KT : Constant  Value=(1.38e-23)*(300)
  Manual Switch : ManualSwitch  CurrentSetting=0
  Product : Product  Inputs=3
  Random Number : RandomNumber  SampleTime=0.1
  Sqrt : Sqrt
  Zero-Order Hold : ZeroOrderHold  SampleTime=1/(2e3*128)
  Out1 : Outport
  wires:
  Product/1 -> Out1/1
  Random Number/1 -> Zero-Order Hold/1
  KT/1 -> 2/Cin/1
  2/Cin/1 -> Sqrt/1
  Constant1/1 -> Manual Switch/2
  Constant/1 -> Manual Switch/1
  Zero-Order Hold/1 -> Product/3
  Sqrt/1 -> Product/2
  Manual Switch/1 -> Product/1

== system dt_crff2_non_ideal/CRFF2/NON-IDEAL INTEGRATOR FOR DT/FLICKER/Flicker Filter ==
  U : Inport
  LTI System1 : cstblocks/LTI System  sys=ff_dt  IC=[]  PadeOrder=0
  Y : Outport
  wires:
  LTI System1/1 -> Y/1
  U/1 -> LTI System1/1

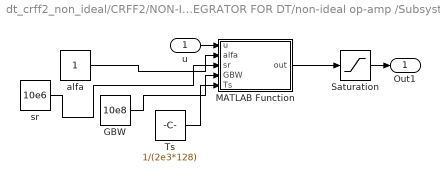
== system dt_crff2_non_ideal/CRFF2/NON-IDEAL INTEGRATOR FOR DT/non-ideal op-amp /Subsystem ==
  u : Inport
  GBW : Constant  Value=10e8
  MATLAB Function : MATLAB Function  TreatAsAtomicUnit=on
  Saturation : Saturate  UpperLimit=0.7  LowerLimit=-0.7
  Ts : Constant  Value=1/(2e3*128)
  alfa : Constant
  sr : Constant  Value=10e6
  Out1 : Outport
  wires:
  Ts/1 -> MATLAB Function/5(Ts)
  MATLAB Function/1(out) -> Saturation/1
  alfa/1 -> MATLAB Function/2(alfa)
  GBW/1 -> MATLAB Function/4(GBW)
  sr/1 -> MATLAB Function/3(sr)
  Saturation/1 -> Out1/1
  u/1 -> MATLAB Function/1(u)

== matlab function dt_crff2_non_ideal/CRFF2/NON-IDEAL INTEGRATOR FOR DT/non-ideal op-amp /Subsystem/MATLAB Function ==
  data: u input; out output; alfa input; sr input; GBW input; Ts input
function out = slew(u, alfa, sr, GBW, Ts)
% Models the op-amp slew rate for a discrete-time integrator
% u    : input signal amplitude (Vp - Vn)
% alfa : finite gain effect (A0/(1+A0)), ideal op-amp alfa = 1
% sr   : slew rate in V/s
% GBW  : gain-bandwidth of op-amp (Hz)
% Ts   : sample time (s)

tau = 1/(2*pi*GBW);   % time constant
Tmax = Ts/2;           % discrete half-step
slope = alfa * abs(u) / tau;

if slope > sr
    % Op-amp is slewing
    tsl = abs(u)*alfa/sr - tau;   % slewing time
    
    if tsl >= Tmax
        % fully slewing entire half period
        error = abs(u) - sr*Tmax;
    else
        % partial slewing, partial linear region
        texp = Tmax - tsl;
        error = abs(u)*(1-alfa) + (alfa*abs(u) - sr*tsl) * exp(-texp/tau);
    end
    
else
    % Linear region (no slewing)
    texp = Tmax;
    error = abs(u)*(1-alfa) + alfa*abs(u)*exp(-texp/tau);
end

out = u - sign(u)*error;
